simulink library "test_IO_log_lib"  (R2018b)
settings: Solver=VariableStepAuto  StartTime=0.0  StopTime=10.0  RelTol=1e-3
settings Model: Creator=taylorreynolds  LastModifiedBy=taylorreynolds

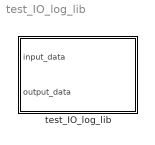
== system test_IO_log_lib ==
  test_IO_log_lib : Subsystem  StopFcn=|  mask{iString1="input_name1", iString2="ignore", iString3="ignore", iString4="ignore", iString5="ignore", iString6="ignore", iString7="ignore", iString8="ignore", iString9="ignore", iString10="ignore", oString1="output_name1", oString2="ignore", oString3="ignore", oString4="ignore", oString5="ignore", oString6="ignore", oString7="ignore", oString8="ignore", oString9="ignore", oString10="ignore"}
      | [input_data,input_name,output_data,output_name] = ...
      | setLoggingIO(input_data1,input_data2,...
      | input_data3,input_data4,input_data5,input_data6,...
      | input_data7,input_data8,input_data9,input_data10,...
      | input_name1,input_name2,input_name3,input_name4,...
      | input_name5,input_name6,input_name7,input_name8,...
      | input_name9,input_name10,...
      | output_data1,output_data2,output_data3,output_data4,...
      | output_data5,output_data6,output_data7,output_data8,...
      | output_data9,output_data10,...
      | output_name1,output_name2,output_name3,output_name4,...
      | output_name5,output_name6,output_name7,output_name8,...
      | output_name9,output_name10);
      | createTestTxtFiles(input_data,input_name,output_data,output_name,gcs);
      mask prompts: iString1 "Set input 1 name"; iString2 "Set input 2 name"; iString3 "Set input 3 name"; iString4 "Set input 4 name"; iString5 "Set input 5 name"; iString6 "Set input 6 name"; iString7 "Set input 7 name"; iString8 "Set input 8 name"; iString9 "Set input 9 name"; iString10 "Set input 10 name"; oString1 "Set output 1 name"; oString2 "Set output 2 name"; oString3 "Set output 3 name"; oString4 "Set output 4 name"; oString5 "Set output 5 name"; oString6 "Set output 6 name"; oString7 "Set output 7 name"; oString8 "Set output 8 name"; oString9 "Set output 9 name"; oString10 "Set output 10 name"
      mask TypeOptions iString1: String Constant/String
      mask TypeOptions iString2: String Constant1/String
      mask TypeOptions iString3: String Constant3/String
      mask TypeOptions iString4: String Constant5/String
      mask TypeOptions iString5: String Constant6/String
      mask TypeOptions iString6: String Constant7/String
      mask TypeOptions iString7: String Constant8/String
      mask TypeOptions iString8: String Constant9/String
      mask TypeOptions iString9: String Constant10/String
      mask TypeOptions iString10: String Constant11/String
      mask TypeOptions oString1: String Constant2/String
      mask TypeOptions oString2: String Constant4/String
      mask TypeOptions oString3: String Constant12/String
      mask TypeOptions oString4: String Constant13/String
      mask TypeOptions oString5: String Constant14/String
      mask TypeOptions oString6: String Constant15/String
      mask TypeOptions oString7: String Constant16/String
      mask TypeOptions oString8: String Constant17/String
      mask TypeOptions oString9: String Constant18/String
      mask TypeOptions oString10: String Constant19/String
      mask DialogControl DescGroupVar Prompt: AACT Test IO Data Logger
      mask DialogControl DescTextVar Prompt: Use these fields to set the names of the input and output data signals. All inputs need to be between quotations like: "<sample_name>" The library will ignore a signal if you set the name to "ignore".
      mask DialogControl ParameterGroupVar Prompt: Input Names
      mask DialogControl Container4 Prompt: Output Names

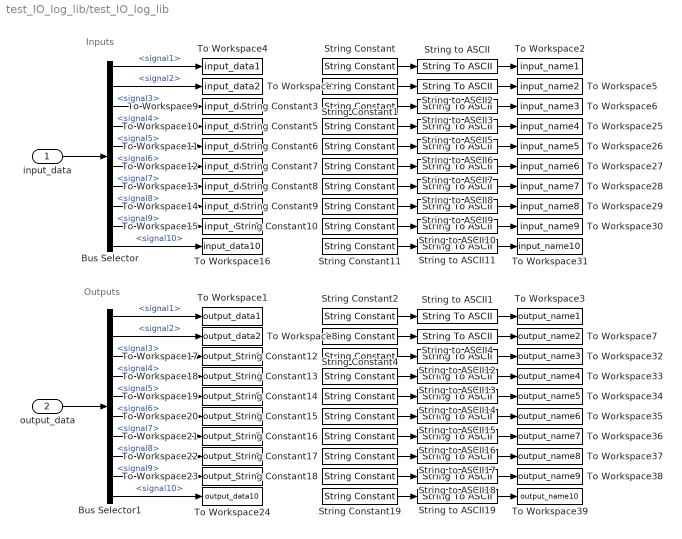
== system test_IO_log_lib/test_IO_log_lib ==
  note: Inputs
  note: Outputs
  input_data : Inport
  output_data : Inport  Port=2
  Bus Selector : BusSelector  OutputSignals=signal1,signal2,signal3,signal4,signal5,signal6,signal7,signal8,signal9,signal10
  Bus Selector1 : BusSelector  OutputSignals=signal1,signal2,signal3,signal4,signal5,signal6,signal7,signal8,signal9,signal10
  String Constant : StringConstant  String=iString1
  String Constant1 : StringConstant  String=iString2
  String Constant10 : StringConstant  String=iString9
  String Constant11 : StringConstant  String=iString10
  String Constant12 : StringConstant  String=oString3
  String Constant13 : StringConstant  String=oString4
  String Constant14 : StringConstant  String=oString5
  String Constant15 : StringConstant  String=oString6
  String Constant16 : StringConstant  String=oString7
  String Constant17 : StringConstant  String=oString8
  String Constant18 : StringConstant  String=oString9
  String Constant19 : StringConstant  String=oString10
  String Constant2 : StringConstant  String=oString1
  String Constant3 : StringConstant  String=iString3
  String Constant4 : StringConstant  String=oString2
  String Constant5 : StringConstant  String=iString4
  String Constant6 : StringConstant  String=iString5
  String Constant7 : StringConstant  String=iString6
  String Constant8 : StringConstant  String=iString7
  String Constant9 : StringConstant  String=iString8
  String to ASCII{,1..19} (20 alike) : StringToASCII
  To Workspace : ToWorkspace  VariableName=input_data2  SampleTime=-1
      settings: Save2DSignal=2-D array (concatenate along first dimension)
  To Workspace1 : ToWorkspace  VariableName=output_data1  SampleTime=-1
      settings: Save2DSignal=2-D array (concatenate along first dimension)
  To Workspace10 : ToWorkspace  VariableName=input_data4  SampleTime=-1
      settings: Save2DSignal=2-D array (concatenate along first dimension)
  To Workspace11 : ToWorkspace  VariableName=input_data5  SampleTime=-1
      settings: Save2DSignal=2-D array (concatenate along first dimension)
  To Workspace12 : ToWorkspace  VariableName=input_data6  SampleTime=-1
      settings: Save2DSignal=2-D array (concatenate along first dimension)
  To Workspace13 : ToWorkspace  VariableName=input_data7  SampleTime=-1
      settings: Save2DSignal=2-D array (concatenate along first dimension)
  To Workspace14 : ToWorkspace  VariableName=input_data8  SampleTime=-1
      settings: Save2DSignal=2-D array (concatenate along first dimension)
  To Workspace15 : ToWorkspace  VariableName=input_data9  SampleTime=-1
      settings: Save2DSignal=2-D array (concatenate along first dimension)
  To Workspace16 : ToWorkspace  VariableName=input_data10  SampleTime=-1
      settings: Save2DSignal=2-D array (concatenate along first dimension)
  To Workspace17 : ToWorkspace  VariableName=output_data3  SampleTime=-1
      settings: Save2DSignal=2-D array (concatenate along first dimension)
  To Workspace18 : ToWorkspace  VariableName=output_data4  SampleTime=-1
      settings: Save2DSignal=2-D array (concatenate along first dimension)
  To Workspace19 : ToWorkspace  VariableName=output_data5  SampleTime=-1
      settings: Save2DSignal=2-D array (concatenate along first dimension)
  To Workspace2 : ToWorkspace  VariableName=input_name1  SampleTime=-1
      settings: MaxDataPoints=1  Save2DSignal=2-D array (concatenate along first dimension)
  To Workspace20 : ToWorkspace  VariableName=output_data6  SampleTime=-1
      settings: Save2DSignal=2-D array (concatenate along first dimension)
  To Workspace21 : ToWorkspace  VariableName=output_data7  SampleTime=-1
      settings: Save2DSignal=2-D array (concatenate along first dimension)
  To Workspace22 : ToWorkspace  VariableName=output_data8  SampleTime=-1
      settings: Save2DSignal=2-D array (concatenate along first dimension)
  To Workspace23 : ToWorkspace  VariableName=output_data9  SampleTime=-1
      settings: Save2DSignal=2-D array (concatenate along first dimension)
  To Workspace24 : ToWorkspace  VariableName=output_data10  SampleTime=-1
      settings: Save2DSignal=2-D array (concatenate along first dimension)
  To Workspace25 : ToWorkspace  VariableName=input_name4  SampleTime=-1
      settings: MaxDataPoints=1  Save2DSignal=2-D array (concatenate along first dimension)
  To Workspace26 : ToWorkspace  VariableName=input_name5  SampleTime=-1
      settings: MaxDataPoints=1  Save2DSignal=2-D array (concatenate along first dimension)
  To Workspace27 : ToWorkspace  VariableName=input_name6  SampleTime=-1
      settings: MaxDataPoints=1  Save2DSignal=2-D array (concatenate along first dimension)
  To Workspace28 : ToWorkspace  VariableName=input_name7  SampleTime=-1
      settings: MaxDataPoints=1  Save2DSignal=2-D array (concatenate along first dimension)
  To Workspace29 : ToWorkspace  VariableName=input_name8  SampleTime=-1
      settings: MaxDataPoints=1  Save2DSignal=2-D array (concatenate along first dimension)
  To Workspace3 : ToWorkspace  VariableName=output_name1  SampleTime=-1
      settings: MaxDataPoints=1  Save2DSignal=2-D array (concatenate along first dimension)
  To Workspace30 : ToWorkspace  VariableName=input_name9  SampleTime=-1
      settings: MaxDataPoints=1  Save2DSignal=2-D array (concatenate along first dimension)
  To Workspace31 : ToWorkspace  VariableName=input_name10  SampleTime=-1
      settings: MaxDataPoints=1  Save2DSignal=2-D array (concatenate along first dimension)
  To Workspace32 : ToWorkspace  VariableName=output_name3  SampleTime=-1
      settings: MaxDataPoints=1  Save2DSignal=2-D array (concatenate along first dimension)
  To Workspace33 : ToWorkspace  VariableName=output_name4  SampleTime=-1
      settings: MaxDataPoints=1  Save2DSignal=2-D array (concatenate along first dimension)
  To Workspace34 : ToWorkspace  VariableName=output_name5  SampleTime=-1
      settings: MaxDataPoints=1  Save2DSignal=2-D array (concatenate along first dimension)
  To Workspace35 : ToWorkspace  VariableName=output_name6  SampleTime=-1
      settings: MaxDataPoints=1  Save2DSignal=2-D array (concatenate along first dimension)
  To Workspace36 : ToWorkspace  VariableName=output_name7  SampleTime=-1
      settings: MaxDataPoints=1  Save2DSignal=2-D array (concatenate along first dimension)
  To Workspace37 : ToWorkspace  VariableName=output_name8  SampleTime=-1
      settings: MaxDataPoints=1  Save2DSignal=2-D array (concatenate along first dimension)
  To Workspace38 : ToWorkspace  VariableName=output_name9  SampleTime=-1
      settings: MaxDataPoints=1  Save2DSignal=2-D array (concatenate along first dimension)
  To Workspace39 : ToWorkspace  VariableName=output_name10  SampleTime=-1
      settings: MaxDataPoints=1  Save2DSignal=2-D array (concatenate along first dimension)
  To Workspace4 : ToWorkspace  VariableName=input_data1  SampleTime=-1
      settings: Save2DSignal=2-D array (concatenate along first dimension)
  To Workspace5 : ToWorkspace  VariableName=input_name2  SampleTime=-1
      settings: MaxDataPoints=1  Save2DSignal=2-D array (concatenate along first dimension)
  To Workspace6 : ToWorkspace  VariableName=input_name3  SampleTime=-1
      settings: MaxDataPoints=1  Save2DSignal=2-D array (concatenate along first dimension)
  To Workspace7 : ToWorkspace  VariableName=output_name2  SampleTime=-1
      settings: MaxDataPoints=1  Save2DSignal=2-D array (concatenate along first dimension)
  To Workspace8 : ToWorkspace  VariableName=output_data2  SampleTime=-1
      settings: Save2DSignal=2-D array (concatenate along first dimension)
  To Workspace9 : ToWorkspace  VariableName=input_data3  SampleTime=-1
      settings: Save2DSignal=2-D array (concatenate along first dimension)
  wires:
  String to ASCII19/1 -> To Workspace39/1
  String Constant19/1 -> String to ASCII19/1
  String Constant18/1 -> String to ASCII18/1
  String to ASCII18/1 -> To Workspace38/1
  String to ASCII17/1 -> To Workspace37/1
  String Constant17/1 -> String to ASCII17/1
  String Constant16/1 -> String to ASCII16/1
  String to ASCII16/1 -> To Workspace36/1
  String to ASCII15/1 -> To Workspace35/1
  String Constant15/1 -> String to ASCII15/1
  String Constant14/1 -> String to ASCII14/1
  String to ASCII14/1 -> To Workspace34/1
  String to ASCII13/1 -> To Workspace33/1
  String Constant13/1 -> String to ASCII13/1
  String Constant12/1 -> String to ASCII12/1
  String to ASCII12/1 -> To Workspace32/1
  String Constant11/1 -> String to ASCII11/1
  String to ASCII11/1 -> To Workspace31/1
  String to ASCII10/1 -> To Workspace30/1
  String Constant10/1 -> String to ASCII10/1
  String Constant9/1 -> String to ASCII9/1
  String to ASCII9/1 -> To Workspace29/1
  String to ASCII8/1 -> To Workspace28/1
  String Constant8/1 -> String to ASCII8/1
  String Constant7/1 -> String to ASCII7/1
  String to ASCII7/1 -> To Workspace27/1
  String to ASCII6/1 -> To Workspace26/1
  String Constant6/1 -> String to ASCII6/1
  String Constant5/1 -> String to ASCII5/1
  String to ASCII5/1 -> To Workspace25/1
  Bus Selector1/10 -> To Workspace24/1  "<signal10>"
  Bus Selector1/9 -> To Workspace23/1  "<signal9>"
  Bus Selector1/8 -> To Workspace22/1  "<signal8>"
  Bus Selector1/7 -> To Workspace21/1  "<signal7>"
  Bus Selector1/6 -> To Workspace20/1  "<signal6>"
  Bus Selector1/5 -> To Workspace19/1  "<signal5>"
  Bus Selector1/4 -> To Workspace18/1  "<signal4>"
  Bus Selector1/3 -> To Workspace17/1  "<signal3>"
  Bus Selector/4 -> To Workspace10/1  "<signal4>"
  Bus Selector/5 -> To Workspace11/1  "<signal5>"
  Bus Selector/6 -> To Workspace12/1  "<signal6>"
  Bus Selector/7 -> To Workspace13/1  "<signal7>"
  Bus Selector/8 -> To Workspace14/1  "<signal8>"
  Bus Selector/9 -> To Workspace15/1  "<signal9>"
  Bus Selector/10 -> To Workspace16/1  "<signal10>"
  Bus Selector1/2 -> To Workspace8/1  "<signal2>"
  output_data/1 -> Bus Selector1/1
  String to ASCII1/1 -> To Workspace3/1
  String Constant2/1 -> String to ASCII1/1
  String to ASCII4/1 -> To Workspace7/1
  Bus Selector1/1 -> To Workspace1/1  "<signal1>"
  String Constant4/1 -> String to ASCII4/1
  String Constant1/1 -> String to ASCII2/1
  input_data/1 -> Bus Selector/1
  String to ASCII2/1 -> To Workspace5/1
  String to ASCII/1 -> To Workspace2/1
  String to ASCII3/1 -> To Workspace6/1
  String Constant3/1 -> String to ASCII3/1
  Bus Selector/2 -> To Workspace/1  "<signal2>"
  Bus Selector/3 -> To Workspace9/1  "<signal3>"
  Bus Selector/1 -> To Workspace4/1  "<signal1>"
  String Constant/1 -> String to ASCII/1
